simulink model "PTCalcModel"  (R2019a)
settings: Solver=FixedStepAuto  StartTime=0.0  StopTime=TimeVectorPT(end)  FixedStep=TsimPT  RelTol=1e-3  EnableMultiTasking=on
undefined symbols (not defined in the file or in its folder): Alt_GIn, P_GOut, T_GIn, T_GOut
libraries: Lib_Solve_ModelSource_TMATS x3, Lib_Turbo_Ambient_TMATS x1
settings Model: Creator=antoniohadadeneto  LastModifiedBy=anton
settings DataIOCC: ReturnWorkspaceOutputs=off
settings OptimizationCC: LifeSpan=inf
settings DebuggingCC: AllowSymbolicDim=off  SFUnexpectedBacktrackingDiag=warning  SFNoUnconditionalDefaultTransitionDiag=warning  SFExecutionAtInitializationDiag=none  ArithmeticOperatorsInVariantConditions=warning
settings ModelReferenceCC: PropagateSignalLabelsOutOfModel=off
settings SFSimCC: SimUseLocalCustomCode=off
settings RTWCC: RTWUseLocalCustomCode=off
settings CodeAppCC: StateflowObjectComments=on
settings GRTTargetCC: TargetLangStandard=C89/C90 (ANSI)
settings ConfigComp: CovMetricSettings=dw  CovHtmlReporting=on  CovSaveCumulativeToWorkspaceVar=on  CovSaveSingleToWorkspaceVar=on  CovExternalEMLEnable=off

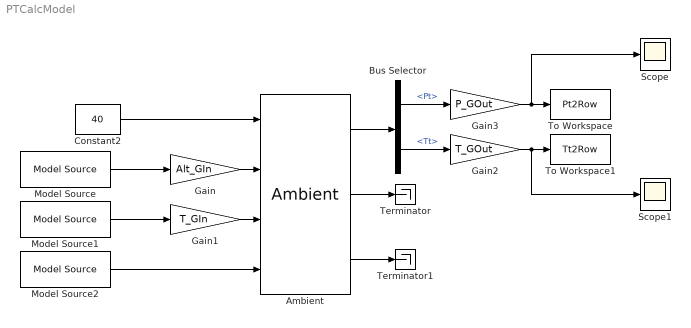
== system PTCalcModel ==
  Ambient : Lib_Turbo_Ambient_TMATS/Ambient  X_A_AltVec_M=5000*[-1 0 1 2 3 4 5 6 7 8 9 10 12 14 16]  T_A_TsVec_M=[536.51 518.67 500.84 483.03 465.22 447.41 429.62 411.84 394.06 389.97 389.97 389.97 389.97 392.25 397.69]  T_A_PsVec_M=[17.554 14.696 12.228 10.108 8.297 6.759 5.461 4.373 3.468 2.73 2.149 1.692 1.049 0.651 0.406]  AFARc_M=0  X_A_FARVec_M=[0; 0.0050; 0.0100; 0.0150; 0.0200; 0.0250; 0.0300]  T_A_RtArray_M="[0.0686;    0.0686;    0.0686;    0.0686;    0.0686;    0.0686;    0.0686]"  Y_A_TVec_M=[300 10000]  T_A_gammaArray_M=[ 1.4 1.4 1.4 1.4 1.4 1.4 1.4; 1.4 1.4 1.4 1.4 1.4 1.4 1.4]
  Bus Selector : BusSelector  OutputSignals=Pt,Tt
  Constant2 : Constant  Value=40
  Gain : Gain  Gain=Alt_GIn
  Gain1 : Gain  Gain=T_GIn
  Gain2 : Gain  Gain=T_GOut
  Gain3 : Gain  Gain=P_GOut
  Model Source : Lib_Solve_ModelSource_TMATS/Model Source  T_vec_M=TimeVectorPT  input_array_M=AltVectorPT
  Model Source1 : Lib_Solve_ModelSource_TMATS/Model Source  T_vec_M=TimeVectorPT  input_array_M=dTVectorPT
  Model Source2 : Lib_Solve_ModelSource_TMATS/Model Source  T_vec_M=TimeVectorPT  input_array_M=MNVectorPT
  Scope : Scope
  Scope1 : Scope
  Terminator : Terminator
  Terminator1 : Terminator
  To Workspace : ToWorkspace  VariableName=Pt2Row  SampleTime=-1
  To Workspace1 : ToWorkspace  VariableName=Tt2Row  SampleTime=-1
  wires:
  Constant2/1 -> Ambient/1
  Bus Selector/2 -> Gain2/1  "<Tt>"
  Ambient/1 -> Bus Selector/1
  Bus Selector/1 -> Gain3/1  "<Pt>"
  Model Source/1 -> Gain/1
  Model Source1/1 -> Gain1/1
  Model Source2/1 -> Ambient/4
  Ambient/2 -> Terminator/1
  Ambient/3 -> Terminator1/1
  Gain/1 -> Ambient/2
  Gain1/1 -> Ambient/3
  Gain2/1 -> Scope1/1, To Workspace1/1
  Gain3/1 -> Scope/1, To Workspace/1
